simulink model "controller_2013B"  (R2013b)
settings: Solver=ode45  StartTime=0.0  StopTime=sim_run  FixedStep=0.001  RelTol=1e-3
InitFcn:
  | zh = 0.01;
undefined symbols (not defined in the file): DiscIntNeverNeededParam, Standard_Devices, UDP_Protocol, zh_step
libraries: rtwinlib x2, simulink x1
settings Model: Creator=Lenka  LastModifiedBy=Anony
settings DebuggingCC: UnderspecifiedInitializationDetection=Simplified  MergeDetectMultiDrivingBlocksExec=error  FrameProcessingCompatibilityMsg=error
settings GRTTargetCC: CodeReplacementLibrary=C89/C90 (ANSI)

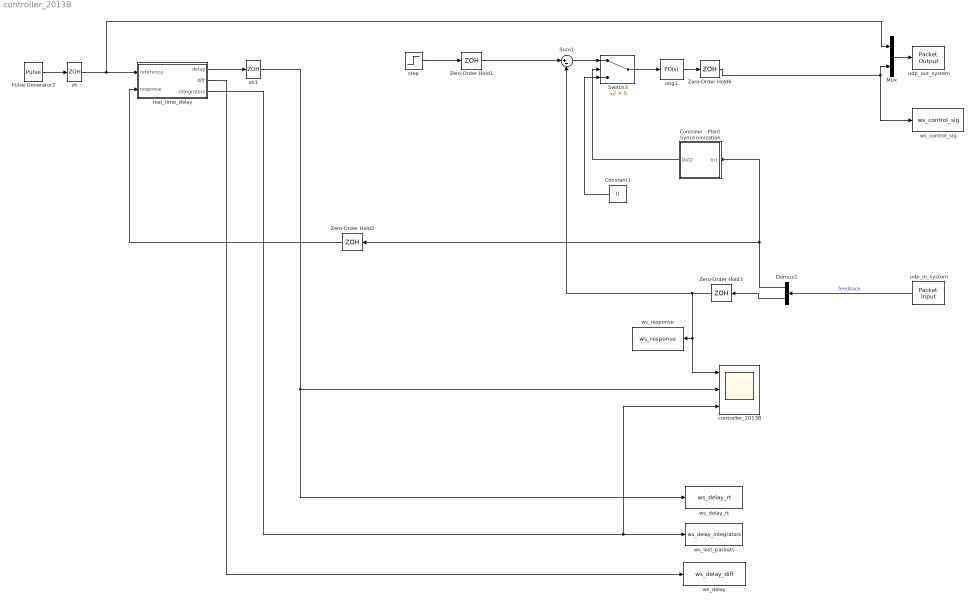
== system controller_2013B ==
  Constant1 : Constant  Value=0  SampleTime=zh_step
  Controler - Plant Synchronization : Subsystem
  Demux1 : Demux  Outputs=2
  Mux : Mux  Inputs=2
  Pulse Generator2 : DiscretePulseGenerator  PulseType=Time based  Period=0.1
  Sum1 : Sum  Inputs=|+-
  Switch3 : Switch  Criteria=u2 > Threshold
  Zero-Order Hold{1..3,6} (4 alike) : ZeroOrderHold  SampleTime=zh_step
  controller_2013B : Scope  NumInputPorts=3
      settings: TimeRange=auto  MaxDataPoints=5000  SaveToWorkspace=off  YMin=-0.00604~-0.01~-0.90875  YMax=0.05439~0.09~8.17875  SampleTime=-1
  orig1 : simulink/Continuous/PID Controller  Controller=PD  TimeDomain=Continuous-time  SampleTime=-1  IntegratorMethod=Forward Euler  FilterMethod=Forward Euler  Form=Parallel  UseFilter=on  ControllerParametersSource=internal  P=0.0142  I=0.0175856984919557  D=0.0001  N=100  InitialConditionSource=internal  InitialConditionForIntegrator=0  InitialConditionForFilter=0  ExternalReset=none  LimitOutput=on  UpperSaturationLimit=5/1000  LowerSaturationLimit=-5/1000  LinearizeAsGain=on  AntiWindupMode=none  Kb=1  TrackingMode=off  Kt=1  PParamMin=[]  PParamMax=[]  IParamMin=[]  IParamMax=[]  DParamMin=[]  DParamMax=[]  NParamMin=[]  NParamMax=[]  KbParamMin=[]  KbParamMax=[]  KtParamMin=[]  KtParamMax=[]  POutMin=[]  POutMax=[]  IOutMin=[]  IOutMax=[]  DOutMin=[]  DOutMax=[]  NOutMin=[]  NOutMax=[]  KbOutMin=[]  KbOutMax=[]  KtOutMin=[]  KtOutMax=[]  IntegratorOutMin=[]  IntegratorOutMax=[]  FilterOutMin=[]  FilterOutMax=[]  SumOutMin=[]  SumOutMax=[]  SumI1OutMin=[]  SumI1OutMax=[]  SumI2OutMin=[]  SumI2OutMax=[]  SumI3OutMin=[]  SumI3OutMax=[]  SumDOutMin=[]  SumDOutMax=[]  SaturationOutMin=[]  SaturationOutMax=[]  IntegratorContinuousStateAttributes=''  IntegratorStateMustResolveToSignalObject=off  IntegratorRTWStateStorageClass=Auto  FilterContinuousStateAttributes=''  FilterStateMustResolveToSignalObject=off  FilterRTWStateStorageClass=Auto  DifferentiatorICPrevScaledInput=0  DifferentiatorOutMin=[]  DifferentiatorOutMax=[]
  real_time_delay : Subsystem
  step : Step  After=0.15  SampleTime=0
  udp_in_system : rtwinlib/Packet Input  SampleTime=0.001  MaxMissedTicks=inf  ShowMissedTicks=off  YieldWhenWaiting=off  DrvName=Standard_Devices/UDP_Protocol  DrvAddress=28500  DrvOptions=[2468394756 28500]  PacketSize=16  DataTypes='2*double'  ShowReady=off  ShowError=off  PacketID=1  ByteOrder=1  ShowTimestamp=off
      settings: AttributesFormatString=Standard Devices\nUDP Protocol [6F5Eh]
  udp_out_system : rtwinlib/Packet Output  SampleTime=0.01  MaxMissedTicks=inf  ShowMissedTicks=off  YieldWhenWaiting=off  DrvName=Standard_Devices/UDP_Protocol  DrvAddress=27500  DrvOptions=[2468394756 27500]  PacketSize=16  DataTypes='2*double'  ShowReady=off  ShowError=off  PacketID=1  ByteOrder=1  InitialValue=[]  FinalValue=[]
      settings: AttributesFormatString=Standard Devices\nUDP Protocol [6B76h]
  ws_control_sig : ToWorkspace  VariableName=ws_control_sig  SaveFormat=Timeseries  SampleTime=zh_step
  ws_delay : ToWorkspace  VariableName=ws_delay_diff  SaveFormat=Timeseries  SampleTime=zh_step
  ws_delay_rt : ToWorkspace  VariableName=ws_delay_rt  SaveFormat=Timeseries  SampleTime=zh_step
  ws_lost_packets : ToWorkspace  VariableName=ws_delay_integrators  SaveFormat=Timeseries  SampleTime=zh_step
  ws_response : ToWorkspace  VariableName=ws_response  SaveFormat=Timeseries  SampleTime=zh_step
  zh : ZeroOrderHold  SampleTime=zh_step
  zh1 : ZeroOrderHold  SampleTime=zh_step
  wires:
  step/1 -> Zero-Order Hold1/1
  Zero-Order Hold1/1 -> Sum1/1
  orig1/1 -> Zero-Order Hold6/1
  zh/1 -> Mux/1, real_time_delay/1(reference)
  Demux1/2 -> Zero-Order Hold3/1
  Mux/1 -> udp_out_system/1
  Zero-Order Hold6/1 -> Mux/2, ws_control_sig/1
  Demux1/1 -> Controler - Plant Synchronization/1(In1), Zero-Order Hold2/1
  udp_in_system/1 -> Demux1/1  "feedback"
  Zero-Order Hold3/1 -> controller_2013B/1, ws_response/1, Sum1/2
  Sum1/1 -> Switch3/1
  Switch3/1 -> orig1/1
  Controler - Plant Synchronization/1(Out2) -> Switch3/2
  Constant1/1 -> Switch3/3
  real_time_delay/1(delay) -> zh1/1
  Pulse Generator2/1 -> zh/1
  Zero-Order Hold2/1 -> real_time_delay/2(response)
  zh1/1 -> ws_delay_rt/1, controller_2013B/2
  real_time_delay/2("diff ") -> ws_delay/1
  real_time_delay/3(integrators) -> controller_2013B/3, ws_lost_packets/1

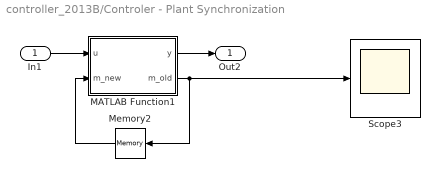
== system controller_2013B/Controler - Plant Synchronization ==
  In1 : Inport
  MATLAB Function1 : MATLAB Function  TreatAsAtomicUnit=on
      settings: PermitHierarchicalResolution=ParametersOnly
  Memory2 : Memory
  Scope3 : Scope
      settings: TimeRange=auto  MaxDataPoints=5000  SaveToWorkspace=off  SaveName=ScopeData2  YMin=-75.00000  YMax=675.00000  SampleTime=-1
  Out2 : Outport
  wires:
  MATLAB Function1/2(m_old) -> Memory2/1, Scope3/1
  Memory2/1 -> MATLAB Function1/2(m_new)
  In1/1 -> MATLAB Function1/1(u)
  MATLAB Function1/1(y) -> Out2/1

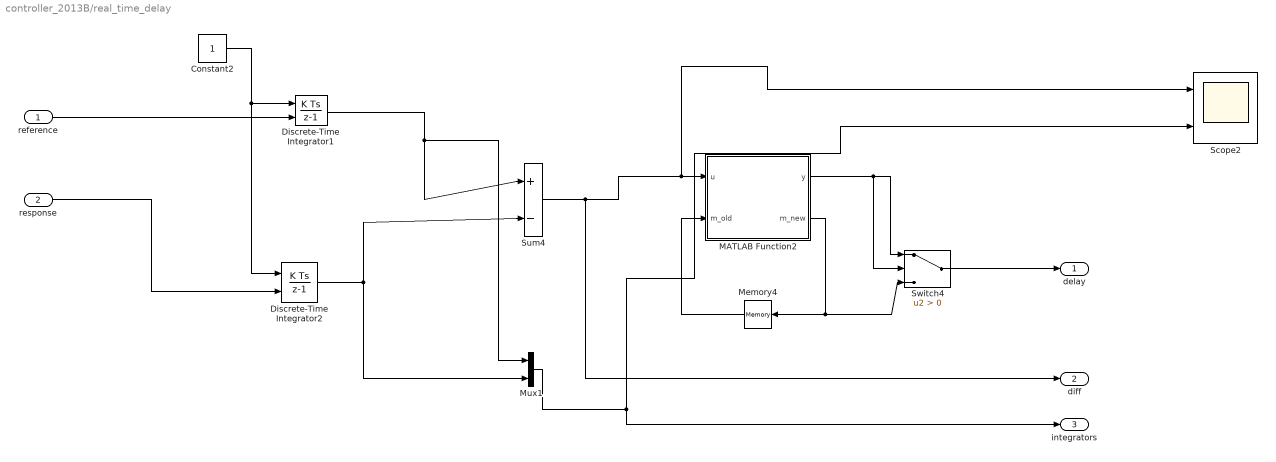
== system controller_2013B/real_time_delay ==
  reference : Inport
  response : Inport  Port=2
  Constant2 : Constant
  Discrete-Time Integrator1 : DiscreteIntegrator  ExternalReset=rising  InitialConditionMode=State only (most efficient)  SampleTime=zh_step  ICPrevOutput=DiscIntNeverNeededParam  ICPrevScaledInput=DiscIntNeverNeededParam
  Discrete-Time Integrator2 : DiscreteIntegrator  ExternalReset=rising  InitialConditionMode=State only (most efficient)  SampleTime=zh_step  ICPrevOutput=DiscIntNeverNeededParam  ICPrevScaledInput=DiscIntNeverNeededParam
  MATLAB Function2 : MATLAB Function  TreatAsAtomicUnit=on
      settings: PermitHierarchicalResolution=ParametersOnly
  Memory4 : Memory
  Mux1 : Mux  Inputs=2
  Scope2 : Scope  NumInputPorts=2
      settings: TimeRange=auto  MaxDataPoints=5000  SaveToWorkspace=off  YMin=-1.6425~-0.1925  YMax=0.2825~1.7325  SampleTime=-1
  Sum4 : Sum  Inputs=|+-
  Switch4 : Switch  Criteria=u2 > Threshold
  delay : Outport
  "diff " : Outport  Port=2
  integrators : Outport  Port=3
  wires:
  Discrete-Time Integrator1/1 -> Mux1/1, Sum4/1
  reference/1 -> Discrete-Time Integrator1/2
  Constant2/1 -> Discrete-Time Integrator2/1, Discrete-Time Integrator1/1
  response/1 -> Discrete-Time Integrator2/2
  Switch4/1 -> delay/1
  MATLAB Function2/2(m_new) -> Memory4/1, Switch4/3
  Memory4/1 -> MATLAB Function2/2(m_old)
  Discrete-Time Integrator2/1 -> Mux1/2, Sum4/2
  MATLAB Function2/1(y) -> Switch4/2, Switch4/1
  Sum4/1 -> "diff "/1, Scope2/1, MATLAB Function2/1(u)
  Mux1/1 -> Scope2/2, integrators/1

== matlab function controller_2013B/Controler - Plant Synchronization/MATLAB Function1 ==
  data: u input; y output; m_new input; m_old output
function [y, m_old] = fcn(u, m_new)
%#codegen

threshold = 600;

if(u > 0 && m_new < threshold)
    m_old = m_new + 1;
else
    m_old = m_new;
end

if(m_old == threshold)
    y = 1;
else
    y=0;
end

== matlab function controller_2013B/real_time_delay/MATLAB Function2 ==
  data: u input; y output; m_new output; m_old input
function [y,m_new] = fcn(u,m_old)
%#codegen
if(u>0)
    y = u;
    m_new = u;
else
    y =0;
    m_new = m_old;
end
